simulink model "Closed_loop_BPS_LQR_Controller"  (R2023b)
settings: Solver=VariableStepAuto  StartTime=0.0  StopTime=3  RelTol=1e-3
undefined symbols (not defined in the file): A, B, C, Continuous, Ke, Kr, Time
libraries: ctrlSharedLib x1
settings Model: Creator=msdbg  LastModifiedBy=msdbg

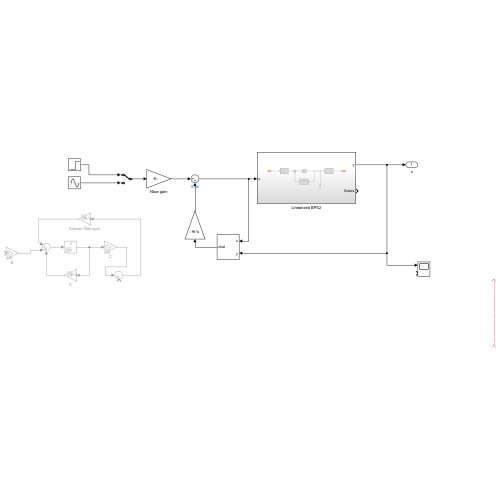
[thumbnail: Simulink's stored preview of the top-level diagram]
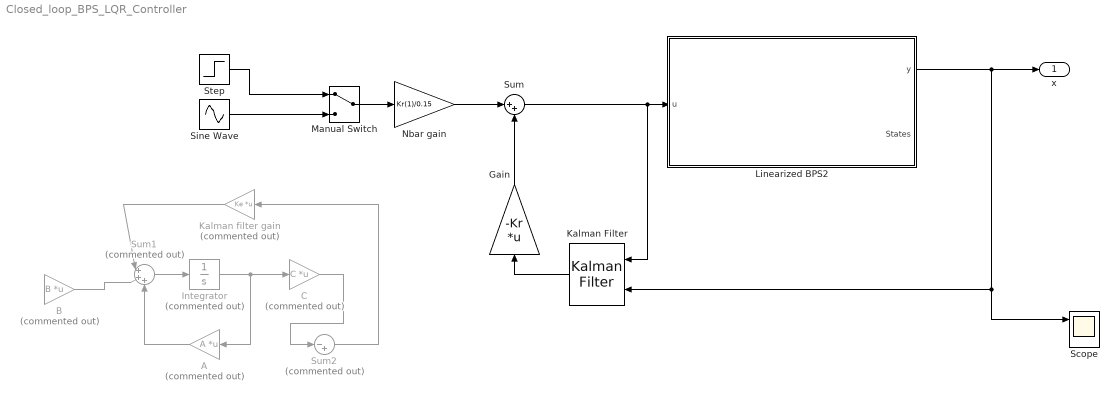
== system Closed_loop_BPS_LQR_Controller ==
  A : Gain  Commented=on  Gain=A  Multiplication=Matrix(K*u)
  B : Gain  Commented=on  Gain=B  Multiplication=Matrix(K*u)
  C : Gain  Commented=on  Gain=C  Multiplication=Matrix(K*u)
  Gain : Gain  Gain=-Kr  Multiplication=Matrix(K*u)
  Integrator : Integrator  Commented=on
  Kalman Filter : ctrlSharedLib/Kalman Filter  TimeDomain=Continuous-Time  UseCurrentEstimator=on  ModelSource=LTI State-Space Variable  ModelSourceVariable=BPS  A=0.95  B=1  C=1  D=0  NumberOfStates=1  NumberOfInputs=1  NumberOfOutputs=1  InitialEstimateSource=Dialog  X0=0  P0=10  UseK=off  UseGH=off  NumberOfProcessNoiseInputs=1  G=1  TimeInvariantG=on  H=0  TimeInvariantH=on  Q=w  TimeInvariantQ=on  R=0.01  TimeInvariantR=on  N=0  TimeInvariantN=on  AddInputPort=on  AddEnablePort=off  OutputEstimatedY=off  OutputP=off  Ts=-1
  Kalman filter gain : Gain  Commented=on  Gain=Ke  Multiplication=Matrix(K*u)
  Linearized BPS2 : Subsystem
  Manual Switch : ManualSwitch
  Nbar gain : Gain  Gain=Kr(1)/0.15
  Scope : Scope  NumInputPorts=2
  Sine Wave : Sin  SampleTime=0
  Step : Step  Time=0  SampleTime=0
  Sum : Sum  Inputs=|++
  Sum1 : Sum  Commented=on  Inputs=|+++
  Sum2 : Sum  Commented=on  Inputs=|-+
  x : Outport
  wires:
  ? -> ?
  Kalman Filter/1 -> Gain/1
  Nbar gain/1 -> Sum/1
  Step/1 -> Manual Switch/1
  Kalman filter gain/1 -> Sum1/1
  C/1 -> Sum2/1
  Sine Wave/1 -> Manual Switch/2
  Manual Switch/1 -> Nbar gain/1
  Gain/1 -> Sum/2
  Integrator/1 -> A/1, C/1
  Sum2/1 -> Kalman filter gain/1
  B/1 -> Sum1/2
  A/1 -> Sum1/3
  Sum1/1 -> Integrator/1
  Sum/1 -> Linearized BPS2/1(u), Kalman Filter/1
  Linearized BPS2/1(y) -> x/1, Scope/1, Kalman Filter/2

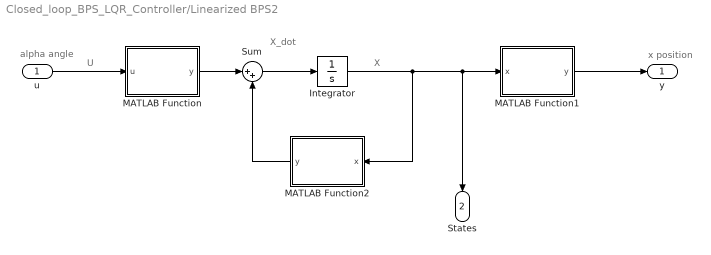
== system Closed_loop_BPS_LQR_Controller/Linearized BPS2 ==
  note: x position
  note: alpha angle
  note: X
  note: X_dot
  note: U
  u : Inport
  Integrator : Integrator
  MATLAB Function : MATLAB Function  TreatAsAtomicUnit=on
  MATLAB Function1 : MATLAB Function  TreatAsAtomicUnit=on
  MATLAB Function2 : MATLAB Function  TreatAsAtomicUnit=on
  Sum : Sum  Inputs=|++
  y : Outport
  States : Outport  Port=2
  wires:
  Sum/1 -> Integrator/1
  Integrator/1 -> MATLAB Function2/1(x), States/1, MATLAB Function1/1(x)
  MATLAB Function/1(y) -> Sum/1
  u/1 -> MATLAB Function/1(u)
  MATLAB Function2/1(y) -> Sum/2
  MATLAB Function1/1(y) -> y/1

== matlab function Closed_loop_BPS_LQR_Controller/Linearized BPS2/MATLAB Function1 ==
  data: x input size=[4 1]; y output
function y = C(x)

y = [1 0 0 0]*x;

== matlab function Closed_loop_BPS_LQR_Controller/Linearized BPS2/MATLAB Function2 ==
  data: x input size=[4 1]; y output size=[4 1]
function y = A(x)

y = [0 1 0 0; 0 0 -5/7*9.81 0; 0 0 0 1; 0 0 -225.4 -22.33]*x;

== matlab function Closed_loop_BPS_LQR_Controller/Linearized BPS2/MATLAB Function ==
  data: u input; y output
function y = B(u)

y = [0; 0; 0; 225.4].*u;
